simulink model "ROSiiwaScratch"  (R2016a)
settings: Solver=FixedStepAuto  StartTime=0.0  StopTime=inf  FixedStep=0.01  RelTol=1e-3
values from neighbouring files (symbols this model uses):
  dt = 0.15    [genKUKATrajectory.m]
  Href = Ttot    [genKUKATrajectory.m]
undefined symbols (not defined in the file or in its folder): Pose, Stiffness
libraries: robotlib x9, realtime_pacer_lib x2, dspsigops x1
settings Model: Creator=victor  LastModifiedBy=localadmin
settings DataIOCC: LimitDataPoints=on
settings OptimizationCC: EfficientFloat2IntCast=on
settings DebuggingCC: AllowSymbolicDim=off
settings ModelReferenceCC: PropagateSignalLabelsOutOfModel=off
settings RTWCC: TargetLang=C++  CheckMdlBeforeBuild=Error
settings GRTTargetCC: GeneratePreprocessorConditionals=Use local settings  MultiInstanceERTCode=on  CodeInterfacePackaging=C++ class

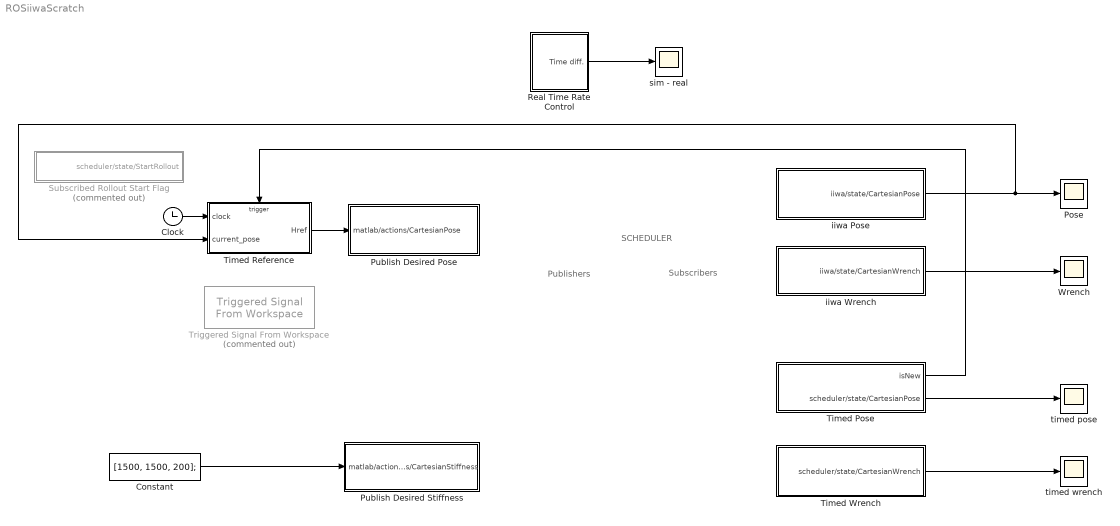
== system ROSiiwaScratch ==
  note: Publishers
  note: Subscribers
  note: SCHEDULER
  Clock : Clock
  Constant : Constant  Value=[1500, 1500, 200];
  Pose : Scope
  Publish Desired Pose : Subsystem
  Publish Desired Stiffness : Subsystem
  Real Time Rate Control : Subsystem
  Subscribed Rollout Start Flag : Subsystem  Commented=on
  Timed Pose : Subsystem
  Timed Wrench : Subsystem
  Timed Reference : Subsystem  TreatAsAtomicUnit=on
  Triggered Signal From Workspace : dspsigops/Triggered Signal From Workspace  Commented=on  Signal=Hd  TriggerType=Rising edge  ic=0  SamplesPerFrame=1  OutputAfterFinalValue=Holding final value  OutputFrames=off
  Wrench : Scope
  iiwa Wrench : Subsystem
  iiwa Pose : Subsystem
  sim - real : Scope
  timed pose : Scope
  timed wrench : Scope
  wires:
  Real Time Rate Control/1(Time diff.) -> sim - real/1
  Constant/1 -> Publish Desired Stiffness/1(" matlab/actions/CartesianStiffness")
  Timed Pose/2(scheduler/state/CartesianPose) -> timed pose/1
  Timed Reference/1(Href) -> Publish Desired Pose/1(matlab/actions/CartesianPose)
  iiwa Wrench/1("iiwa/state/CartesianWrench ") -> Wrench/1
  iiwa Pose/1(iiwa/state/CartesianPose) -> Timed Reference/2(current_pose), Pose/1
  Clock/1 -> Timed Reference/1(clock)
  Timed Pose/1(isNew) -> Timed Reference/Trigger
  Timed Wrench/1(scheduler/state/CartesianWrench) -> timed wrench/1

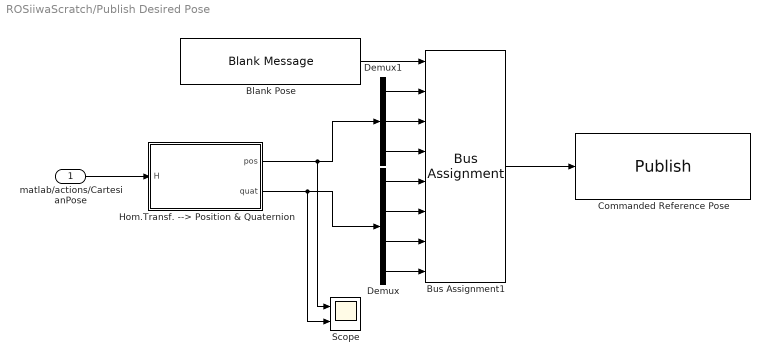
== system ROSiiwaScratch/Publish Desired Pose ==
  matlab/actions/CartesianPose : Inport
  Blank Pose : robotlib/Blank Message  SourceLibraryInfo=This block requires Robotics System Toolbox  messageType=geometry_msgs/PoseStamped  SampleTime=inf
  Bus Assignment1 : BusAssignment  AssignedSignals=Pose.Position.X,Pose.Position.Y,Pose.Position.Z,Pose.Orientation.X,Pose.Orientation.Y,Pose.Orientation.Z,Pose.Orientation.W
  Commanded Reference Pose : robotlib/Publish  SourceLibraryInfo=This block requires Robotics System Toolbox  topicSource=Specify your own  topic=/matlab/actions/CartesianPose  messageType=geometry_msgs/PoseStamped  messageQueueLength=1
  Demux : Demux
  Demux1 : Demux  Outputs=3
  Hom.Transf. --> Position & Quaternion : MATLAB Function  TreatAsAtomicUnit=on
  Scope : Scope  NumInputPorts=2
  wires:
  matlab/actions/CartesianPose/1 -> Hom.Transf. --> Position & Quaternion/1(H)
  Bus Assignment1/1 -> Commanded Reference Pose/1
  Blank Pose/1 -> Bus Assignment1/1
  Demux/1 -> Bus Assignment1/5
  Demux/2 -> Bus Assignment1/6
  Demux/3 -> Bus Assignment1/7
  Demux1/1 -> Bus Assignment1/2
  Demux1/2 -> Bus Assignment1/3
  Demux1/3 -> Bus Assignment1/4
  Hom.Transf. --> Position & Quaternion/1(pos) -> Scope/1, Demux1/1
  Demux/4 -> Bus Assignment1/8
  Hom.Transf. --> Position & Quaternion/2(quat) -> Scope/2, Demux/1

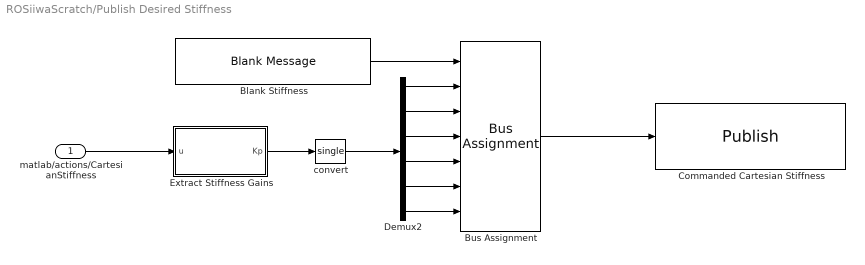
== system ROSiiwaScratch/Publish Desired Stiffness ==
  " matlab/actions/CartesianStiffness" : Inport
  Blank Stiffness : robotlib/Blank Message  SourceLibraryInfo=This block requires Robotics System Toolbox  messageType=iiwa_msgs/CartesianStiffness  SampleTime=inf
  Bus Assignment : BusAssignment  AssignedSignals=Stiffness.X,Stiffness.Y,Stiffness.Z,Stiffness.A,Stiffness.B,Stiffness.C
  Commanded Cartesian Stiffness : robotlib/Publish  SourceLibraryInfo=This block requires Robotics System Toolbox  topicSource=Specify your own  topic=/matlab/actions/CartesianStiffness  messageType=iiwa_msgs/CartesianStiffness  messageQueueLength=1
  Demux2 : Demux  Outputs=6
  Extract Stiffness Gains : MATLAB Function  TreatAsAtomicUnit=on
  convert : DataTypeConversion  OutDataTypeStr=single
  wires:
  Blank Stiffness/1 -> Bus Assignment/1
  Bus Assignment/1 -> Commanded Cartesian Stiffness/1
  Demux2/4 -> Bus Assignment/5
  Demux2/6 -> Bus Assignment/7
  Demux2/5 -> Bus Assignment/6
  Demux2/3 -> Bus Assignment/4
  Demux2/2 -> Bus Assignment/3
  Demux2/1 -> Bus Assignment/2
  " matlab/actions/CartesianStiffness"/1 -> Extract Stiffness Gains/1(u)
  Extract Stiffness Gains/1(Kp) -> convert/1
  convert/1 -> Demux2/1

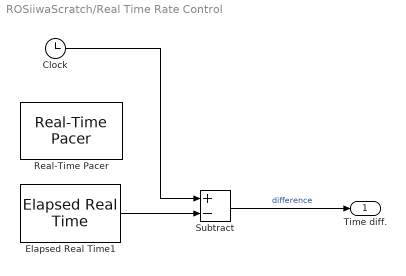
== system ROSiiwaScratch/Real Time Rate Control ==
  Clock : Clock
  Elapsed Real Time1 : realtime_pacer_lib/Elapsed Real Time
  Real-Time Pacer : realtime_pacer_lib/Real-Time Pacer  simTimePerRealTime=1
  Subtract : Sum  Inputs=+-
  Time diff. : Outport
  wires:
  Elapsed Real Time1/1 -> Subtract/2
  Subtract/1 -> Time diff./1  "difference"
  Clock/1 -> Subtract/1

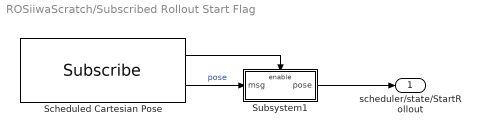
== system ROSiiwaScratch/Subscribed Rollout Start Flag ==
  Scheduled Cartesian Pose : robotlib/Subscribe  SourceLibraryInfo=This block requires Robotics System Toolbox  topicSource=Specify your own  topic=/scheduler/state/StartRollout  messageType=std_msgs/Bool  sampleTime=-1  messageQueueLength=1
  Subsystem1 : Subsystem
  scheduler/state/StartRollout : Outport
  wires:
  Scheduled Cartesian Pose/2 -> Subsystem1/1(msg)  "pose"
  Subsystem1/1(pose) -> scheduler/state/StartRollout/1
  Scheduled Cartesian Pose/1 -> Subsystem1/Enable

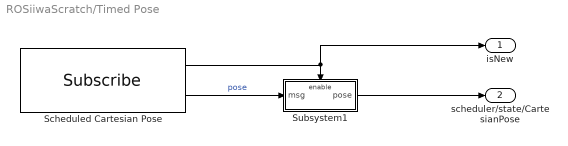
== system ROSiiwaScratch/Timed Pose ==
  Scheduled Cartesian Pose : robotlib/Subscribe  SourceLibraryInfo=This block requires Robotics System Toolbox  topicSource=Specify your own  topic=/scheduler/state/CartesianPose  messageType=geometry_msgs/PoseStamped  sampleTime=-1  messageQueueLength=1
  Subsystem1 : Subsystem
  isNew : Outport
  scheduler/state/CartesianPose : Outport  Port=2
  wires:
  Scheduled Cartesian Pose/2 -> Subsystem1/1(msg)  "pose"
  Subsystem1/1(pose) -> scheduler/state/CartesianPose/1
  Scheduled Cartesian Pose/1 -> isNew/1, Subsystem1/Enable

== system ROSiiwaScratch/Timed Wrench ==
  Scheduled Cartesian Pose : robotlib/Subscribe  SourceLibraryInfo=This block requires Robotics System Toolbox  topicSource=Specify your own  topic=/scheduler/state/CartesianWrench  messageType=geometry_msgs/WrenchStamped  sampleTime=-1  messageQueueLength=1
  Subsystem1 : Subsystem
  scheduler/state/CartesianWrench : Outport
  wires:
  Scheduled Cartesian Pose/2 -> Subsystem1/1(msg)  "pose"
  Subsystem1/1(pose) -> scheduler/state/CartesianWrench/1
  Scheduled Cartesian Pose/1 -> Subsystem1/Enable

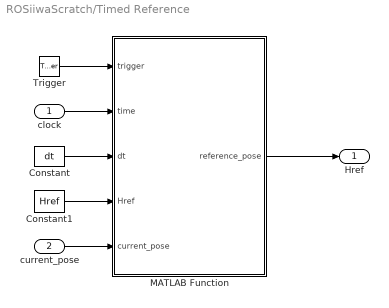
== system ROSiiwaScratch/Timed Reference ==
  clock : Inport
  current_pose : Inport  Port=2
  Trigger : TriggerPort  VariantControl=Variant  ShowOutputPort=on  PortDimensions=1
  Constant : Constant  Value=dt
  Constant1 : Constant  Value=Href
  MATLAB Function : MATLAB Function  TreatAsAtomicUnit=on
  Href : Outport
  wires:
  MATLAB Function/1(reference_pose) -> Href/1
  Trigger/1 -> MATLAB Function/1(trigger)
  clock/1 -> MATLAB Function/2(time)
  current_pose/1 -> MATLAB Function/5(current_pose)
  Constant/1 -> MATLAB Function/3(dt)
  Constant1/1 -> MATLAB Function/4(Href)

== system ROSiiwaScratch/iiwa Wrench ==
  Subsystem2 : Subsystem
  iiwa Cartesian Wrench : robotlib/Subscribe  SourceLibraryInfo=This block requires Robotics System Toolbox  topicSource=Specify your own  topic=/iiwa/state/CartesianWrench  messageType=geometry_msgs/WrenchStamped  sampleTime=-1  messageQueueLength=1
  "iiwa/state/CartesianWrench " : Outport
  wires:
  iiwa Cartesian Wrench/2 -> Subsystem2/1(msg)  "pose"
  iiwa Cartesian Wrench/1 -> Subsystem2/Enable
  Subsystem2/1(wrench) -> "iiwa/state/CartesianWrench "/1

== system ROSiiwaScratch/iiwa Pose ==
  Scheduled Cartesian Pose : robotlib/Subscribe  SourceLibraryInfo=This block requires Robotics System Toolbox  topicSource=Specify your own  topic=/iiwa/state/CartesianPose  messageType=geometry_msgs/PoseStamped  sampleTime=-1  messageQueueLength=1
  Subsystem1 : Subsystem
  iiwa/state/CartesianPose : Outport
  wires:
  Scheduled Cartesian Pose/2 -> Subsystem1/1(msg)  "pose"
  Subsystem1/1(pose) -> iiwa/state/CartesianPose/1
  Scheduled Cartesian Pose/1 -> Subsystem1/Enable

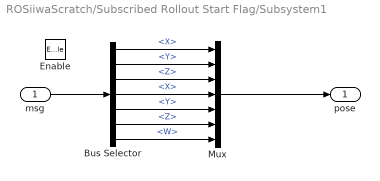
== system ROSiiwaScratch/Subscribed Rollout Start Flag/Subsystem1 ==
  msg : Inport
  Enable : EnablePort
  Bus Selector : BusSelector  OutputSignals=Pose.Position.X,Pose.Position.Y,Pose.Position.Z,Pose.Orientation.X,Pose.Orientation.Y,Pose.Orientation.Z,Pose.Orientation.W
  Mux : Mux  Inputs=7
  pose : Outport
  wires:
  Bus Selector/3 -> Mux/3  "<Z>"
  Bus Selector/1 -> Mux/1  "<X>"
  Bus Selector/2 -> Mux/2  "<Y>"
  Mux/1 -> pose/1
  msg/1 -> Bus Selector/1
  Bus Selector/4 -> Mux/4  "<X>"
  Bus Selector/5 -> Mux/5  "<Y>"
  Bus Selector/6 -> Mux/6  "<Z>"
  Bus Selector/7 -> Mux/7  "<W>"

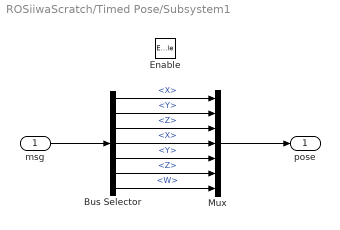
== system ROSiiwaScratch/Timed Pose/Subsystem1 ==
  msg : Inport
  Enable : EnablePort
  Bus Selector : BusSelector  OutputSignals=Pose.Position.X,Pose.Position.Y,Pose.Position.Z,Pose.Orientation.X,Pose.Orientation.Y,Pose.Orientation.Z,Pose.Orientation.W
  Mux : Mux  Inputs=7
  pose : Outport
  wires:
  Bus Selector/3 -> Mux/3  "<Z>"
  Bus Selector/1 -> Mux/1  "<X>"
  Bus Selector/2 -> Mux/2  "<Y>"
  Mux/1 -> pose/1
  msg/1 -> Bus Selector/1
  Bus Selector/4 -> Mux/4  "<X>"
  Bus Selector/5 -> Mux/5  "<Y>"
  Bus Selector/6 -> Mux/6  "<Z>"
  Bus Selector/7 -> Mux/7  "<W>"

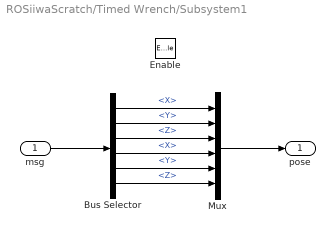
== system ROSiiwaScratch/Timed Wrench/Subsystem1 ==
  msg : Inport
  Enable : EnablePort
  Bus Selector : BusSelector  OutputSignals=Wrench.Force.X,Wrench.Force.Y,Wrench.Force.Z,Wrench.Torque.X,Wrench.Torque.Y,Wrench.Torque.Z
  Mux : Mux  Inputs=6
  pose : Outport
  wires:
  Bus Selector/3 -> Mux/3  "<Z>"
  Bus Selector/1 -> Mux/1  "<X>"
  Bus Selector/2 -> Mux/2  "<Y>"
  Mux/1 -> pose/1
  msg/1 -> Bus Selector/1
  Bus Selector/4 -> Mux/4  "<X>"
  Bus Selector/5 -> Mux/5  "<Y>"
  Bus Selector/6 -> Mux/6  "<Z>"

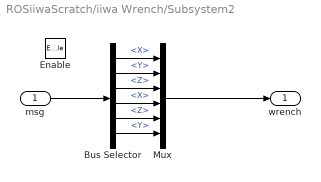
== system ROSiiwaScratch/iiwa Wrench/Subsystem2 ==
  msg : Inport
  Enable : EnablePort
  Bus Selector : BusSelector  OutputSignals=Wrench.Force.X,Wrench.Force.Y,Wrench.Force.Z,Wrench.Torque.X,Wrench.Torque.Z,Wrench.Torque.Y
  Mux : Mux  Inputs=6
  wrench : Outport
  wires:
  Bus Selector/3 -> Mux/3  "<Z>"
  Bus Selector/1 -> Mux/1  "<X>"
  Bus Selector/2 -> Mux/2  "<Y>"
  Mux/1 -> wrench/1
  msg/1 -> Bus Selector/1
  Bus Selector/4 -> Mux/4  "<X>"
  Bus Selector/5 -> Mux/5  "<Z>"
  Bus Selector/6 -> Mux/6  "<Y>"

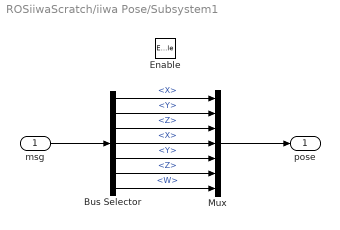
== system ROSiiwaScratch/iiwa Pose/Subsystem1 ==
  msg : Inport
  Enable : EnablePort
  Bus Selector : BusSelector  OutputSignals=Pose.Position.X,Pose.Position.Y,Pose.Position.Z,Pose.Orientation.X,Pose.Orientation.Y,Pose.Orientation.Z,Pose.Orientation.W
  Mux : Mux  Inputs=7
  pose : Outport
  wires:
  Bus Selector/3 -> Mux/3  "<Z>"
  Bus Selector/1 -> Mux/1  "<X>"
  Bus Selector/2 -> Mux/2  "<Y>"
  Mux/1 -> pose/1
  msg/1 -> Bus Selector/1
  Bus Selector/4 -> Mux/4  "<X>"
  Bus Selector/5 -> Mux/5  "<Y>"
  Bus Selector/6 -> Mux/6  "<Z>"
  Bus Selector/7 -> Mux/7  "<W>"

== matlab function ROSiiwaScratch/Publish Desired Pose/Hom.Transf. --> Position & Quaternion ==
  data: H input size=[4 4]; pos output double size=[3 1]; quat output double size=[4 1]
function [pos, quat] = minimRep(H)
%# convert transformation matrix into position vector and quaternion vector

pos = transl(H);    % [x y z]'

quat = tform2quat(H)'; % [w x y z]'

== matlab function ROSiiwaScratch/Publish Desired Stiffness/Extract Stiffness Gains ==
  data: u input size=[3 1]; Kp output double size=[6 1]
function Kp = arrangeGains(u)
%# arranges gains stiffness gains in suitable manner. 
% !! HARD CODED !! change for different scenarios !@!@

Kp = [u(1), u(2), u(2), u(3), u(3), u(3)]';

== matlab function ROSiiwaScratch/Timed Reference/MATLAB Function ==
  data: trigger input; reference_pose output; time input; dt input; Href input; current_pose input
function reference_pose = startReference(trigger, time, dt, Href, current_pose)
% Timed output of the reference homogeneous transform. 
% Monitors a trigger send by the scheduling script to synchronize the
% command reference.
%
% code by Victor van Spaandonk
% July 2016
%% inits
persistent startTime;
if isempty(startTime)
    startTime = 0;
end

T=10;
current_pose
%% code
% set reference to current position:
reference_pose = quat2tform(current_pose(4:end,1)');
reference_pose(1:3,4) = current_pose(1:3,1);

if trigger && startTime==0
    startTime = time;
elseif trigger
    current_time = (time - startTime)/dt
    if current_time < T/dt
        reference_pose = Href(:,:,floor(current_time)+1);   % update reference value
    else 
        reference_pose = Href(:,:,end);                     % hold final value
    end
end
reference_pose
end
